simulink model "testingPLUT"  (R2019b)
settings: Solver=VariableStepAuto  StartTime=0.0  StopTime=stop_time  RelTol=1e-3
values from neighbouring files (symbols this model uses):
  X_in = X_temp    [TestingLibraryScripts.m]
libraries: DSP_FPGA_Accelerated_Toolbox x1
settings Model: Creator=Bailey  LastModifiedBy=Balad
settings SFSimCC: CustomCodeUndefinedFunction=UseInterfaceOnly

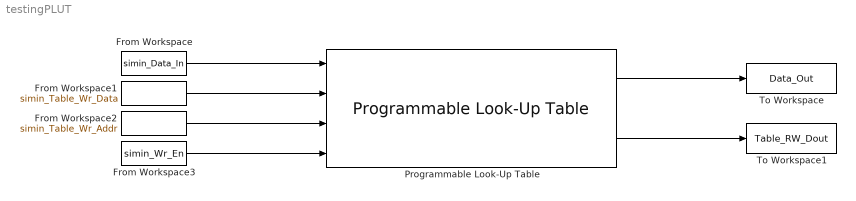
== system testingPLUT ==
  From Workspace : FromWorkspace  VariableName=simin_Data_In  SampleTime=0  Interpolate=off
  From Workspace1 : FromWorkspace  VariableName=simin_Table_Wr_Data  SampleTime=0  Interpolate=off
  From Workspace2 : FromWorkspace  VariableName=simin_Table_Wr_Addr  SampleTime=0  Interpolate=off
  From Workspace3 : FromWorkspace  VariableName=simin_Wr_En  SampleTime=0  Interpolate=off
  Programmable Look-Up Table : DSP_FPGA_Accelerated_Toolbox/Programmable Look-Up Table  TableFn=X_in.^0.5  maxInput=1  floor_in_tab=2^-15  error_cap_tab=0.02  ERR_DIAG=on  N_bits_tab=4  M_bits_tab=5  igotthis=off  Table_Init=0  d=0
      settings: SourceProductName=DSP FPGA Accelerated Toolbox
  To Workspace : ToWorkspace  VariableName=Data_Out  SaveFormat=Timeseries  SampleTime=-1
  To Workspace1 : ToWorkspace  VariableName=Table_RW_Dout  SaveFormat=Timeseries  SampleTime=-1
  wires:
  Programmable Look-Up Table/1 -> To Workspace/1
  Programmable Look-Up Table/2 -> To Workspace1/1
  From Workspace/1 -> Programmable Look-Up Table/1
  From Workspace3/1 -> Programmable Look-Up Table/4
  From Workspace2/1 -> Programmable Look-Up Table/3
  From Workspace1/1 -> Programmable Look-Up Table/2
